simulink model "RZPOLLAR"  (R2015a)
settings: Solver=ode45  StartTime=0.0  StopTime=100  RelTol=1e-3
libraries: commrandsrc2 x1, simulink_extras x1
settings Model: Creator=user  LastModifiedBy=user

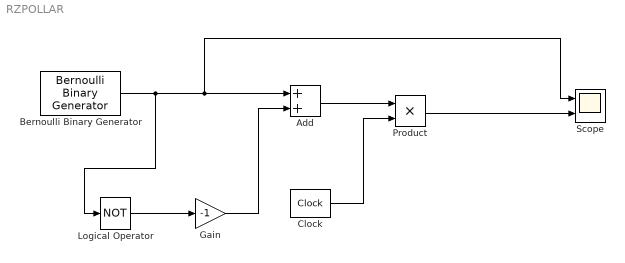
== system RZPOLLAR ==
  Add : Sum
  Bernoulli Binary Generator : commrandsrc2/Bernoulli Binary Generator  P=0.5  seed=61  Ts=0.5  frameBased=off  sampPerFrame=1  orient=off  outDataType=double
  Clock : simulink_extras/Flip Flops/Clock  period=2
  Gain : Gain  Gain=-1
  Logical Operator : Logic  Operator=NOT  AllPortsSameDT=off  OutDataTypeStr=boolean
  Product : Product
  Scope : Scope  NumInputPorts=2
      settings: YMin=-5~-5  YMax=5~5
  wires:
  Logical Operator/1 -> Gain/1
  Bernoulli Binary Generator/1 -> Logical Operator/1, Scope/1, Add/1
  Gain/1 -> Add/2
  Clock/1 -> Product/2
  Add/1 -> Product/1
  Product/1 -> Scope/2
